simulink model "SR"  (R2014a)
settings: Solver=ode45  StartTime=0.0  StopTime=0.4  RelTol=1e-3
settings Model: Creator=User  LastModifiedBy=Анастасия

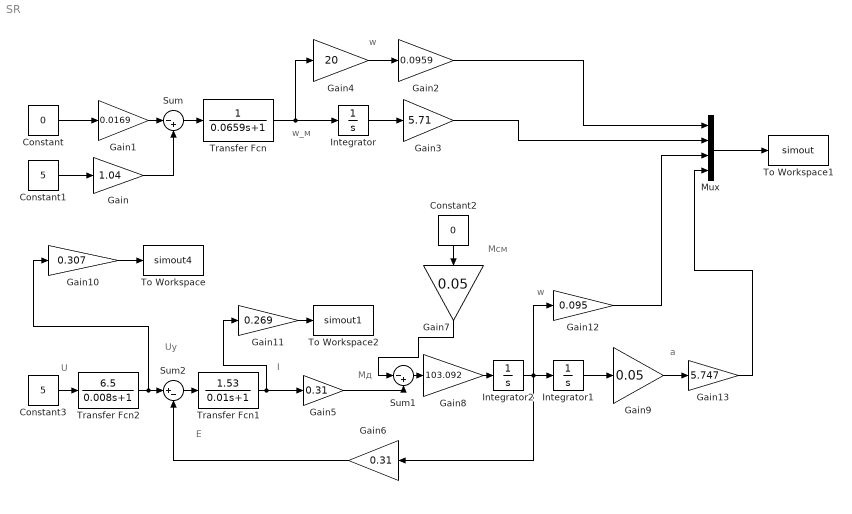
== system SR ==
  note: w
  note: w_м
  note: E
  note: a
  note: w
  note: Мд
  note: Mсм
  note: I
  note: Uy
  note: U
  Constant : Constant  Value=0
  Constant1 : Constant  Value=5
  Constant2 : Constant  Value=0
  Constant3 : Constant  Value=5
  Gain : Gain  Gain=1.04
  Gain1 : Gain  Gain=0.0169
  Gain10 : Gain  Gain=0.307
  Gain11 : Gain  Gain=0.269
  Gain12 : Gain  Gain=0.095
  Gain13 : Gain  Gain=5.747
  Gain2 : Gain  Gain=0.0959
  Gain3 : Gain  Gain=5.71
  Gain4 : Gain  Gain=20
  Gain5 : Gain  Gain=0.31
  Gain6 : Gain  Gain=0.31
  Gain7 : Gain  Gain=0.05
  Gain8 : Gain  Gain=103.092
  Gain9 : Gain  Gain=0.05
  Integrator : Integrator
  Integrator1 : Integrator
  Integrator2 : Integrator
  Mux : Mux
  Sum : Sum  Inputs=|-+
  Sum1 : Sum  Inputs=|-+
  Sum2 : Sum  Inputs=|+-
  To Workspace : ToWorkspace  VariableName=simout4  SaveFormat=Timeseries  SampleTime=-1
  To Workspace1 : ToWorkspace  VariableName=simout  SaveFormat=Timeseries  SampleTime=-1
  To Workspace2 : ToWorkspace  VariableName=simout1  SaveFormat=Timeseries  SampleTime=-1
  Transfer Fcn : TransferFcn  Denominator=[0.0659 1]
  Transfer Fcn1 : TransferFcn  Numerator=[1.53]  Denominator=[0.01 1]
  Transfer Fcn2 : TransferFcn  Numerator=[6.5]  Denominator=[0.008 1]
  wires:
  Sum/1 -> Transfer Fcn/1
  Integrator/1 -> Gain3/1
  Constant1/1 -> Gain/1
  Constant/1 -> Gain1/1
  Gain/1 -> Sum/2
  Gain1/1 -> Sum/1
  Transfer Fcn/1 -> Integrator/1, Gain4/1
  Gain2/1 -> Mux/1
  Gain3/1 -> Mux/2
  Gain4/1 -> Gain2/1
  Constant3/1 -> Transfer Fcn2/1
  Transfer Fcn2/1 -> Gain10/1, Sum2/1
  Transfer Fcn1/1 -> Gain11/1, Gain5/1
  Gain5/1 -> Sum1/2
  Constant2/1 -> Gain7/1
  Gain7/1 -> Sum1/1
  Sum1/1 -> Gain8/1
  Gain8/1 -> Integrator2/1
  Integrator2/1 -> Gain12/1, Gain6/1, Integrator1/1
  Gain6/1 -> Sum2/2
  Sum2/1 -> Transfer Fcn1/1
  Integrator1/1 -> Gain9/1
  Gain9/1 -> Gain13/1
  Gain13/1 -> Mux/4
  Gain12/1 -> Mux/3
  Gain11/1 -> To Workspace2/1
  Gain10/1 -> To Workspace/1
  Mux/1 -> To Workspace1/1
